simulink model "Mondmission"  (R2014b)
settings: Solver=ode45  StartTime=0.0  StopTime=2000000  RelTol=1e-3
settings Model: Creator=hollowman  LastModifiedBy=sigurd

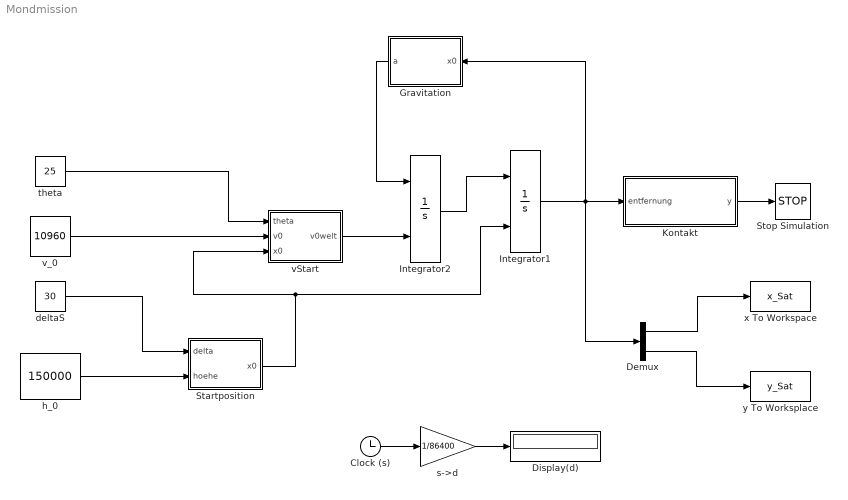
== system Mondmission ==
  Clock (s) : Clock
  Demux : Demux  Outputs=2
  Display(d) : Display
  Gravitation : MATLAB Function  TreatAsAtomicUnit=on
  Integrator1 : Integrator  InitialConditionSource=external
  Integrator2 : Integrator  InitialConditionSource=external
  Kontakt : MATLAB Function  TreatAsAtomicUnit=on
  Startposition : MATLAB Function  TreatAsAtomicUnit=on
  Stop Simulation : Stop
  deltaS : Constant  Value=30
  h_0 : Constant  Value=150000
  s->d : Gain  Gain=1/86400
  theta : Constant  Value=25
  vStart : MATLAB Function  TreatAsAtomicUnit=on
  v_0 : Constant  Value=10960
  x To Workspace : ToWorkspace  VariableName=x_Sat  SampleTime=-1
  y To Worksplace : ToWorkspace  VariableName=y_Sat  SampleTime=-1
  wires:
  Clock (s)/1 -> s->d/1
  s->d/1 -> Display(d)/1
  Demux/1 -> x To Workspace/1
  Demux/2 -> y To Worksplace/1
  Kontakt/1(y) -> Stop Simulation/1
  h_0/1 -> Startposition/2(hoehe)
  deltaS/1 -> Startposition/1(delta)
  Startposition/1(x0) -> vStart/3(x0), Integrator1/2
  theta/1 -> vStart/1(theta)
  v_0/1 -> vStart/2(v0)
  Integrator1/1 -> Gravitation/1(x0), Demux/1, Kontakt/1(entfernung)
  vStart/1(v0welt) -> Integrator2/2
  Gravitation/1(a) -> Integrator2/1
  Integrator2/1 -> Integrator1/1

== matlab function Mondmission/Startposition ==
  data: delta input; x0 output; hoehe input
function x0 = fcn(delta, hoehe)
er = 6378000; % Erdradius in Meter
bogen_delta = delta * pi() / 180;
x  = cos(bogen_delta) * (er + hoehe); 
y  = sin(bogen_delta) * (er + hoehe);
% Startposition als Spaltenvektor
x0 = [x ; y]

== matlab function Mondmission/vStart ==
  data: theta input; v0 input; x0 input; v0welt output
function v0welt = fcn(theta, v0, x0)

bogen_theta = theta * pi / 180;

normE = x0 / norm(x0);              % Einheitsvektor in Normalrichtung
tanE = [normE(2) ; -normE(1)];      % Einheitvektor in Tangentialrichtung

t = cos(bogen_theta) * v0;          % Tangentialkomponente
n = sin(bogen_theta) * v0;          % Normalkomponente

v0welt = (t * tanE) + (n * normE);  % Geschwindigkeitsvektor

== matlab function Mondmission/Gravitation ==
  data: x0 input; a output
function a = fcn(x0)

G = 66.743 * 10^(-12); % Gravitationskonstante
m_Erde = 5.9736 * 10^24; % Masse der Erde

x_Mond = [0 ; -380000000] % Position des Monds
m_Mond = 7.3480 * 10^22; % Masse des Mondes

v_Mond =  x0 - x_Mond; % Vektor Sat richtung Mond

r_Erde = norm(x0); % Entfernung zur Erde
r_Mond = norm(v_Mond); % Entfernung zum Mond

richtungE = -x0 / r_Erde; % Einheitsvektor Erde-Satelit
richtungM = -v_Mond / r_Mond; % Einheitsvektor Mond-Satelit

a_Mond = richtungM * G * m_Mond / r_Mond^2
a = (richtungE * G * m_Erde / r_Erde^2) + a_Mond; % Gravitationsbeschl.

== matlab function Mondmission/Kontakt ==
  data: entfernung input; y output
function y = fcn(entfernung)
entfernung = norm(entfernung);

if(entfernung<=6378000)
    y = 1;
else
    y = 0;
end;
